simulink model "test_transfer_function"  (R2019b)
settings: Solver=ode4  StartTime=0.0  StopTime=100  FixedStep=1e-3  RelTol=1e-3
libraries: simulink x1
settings Model: Creator=bitgar  LastModifiedBy=bitgar
settings DataIOCC: ReturnWorkspaceOutputs=off

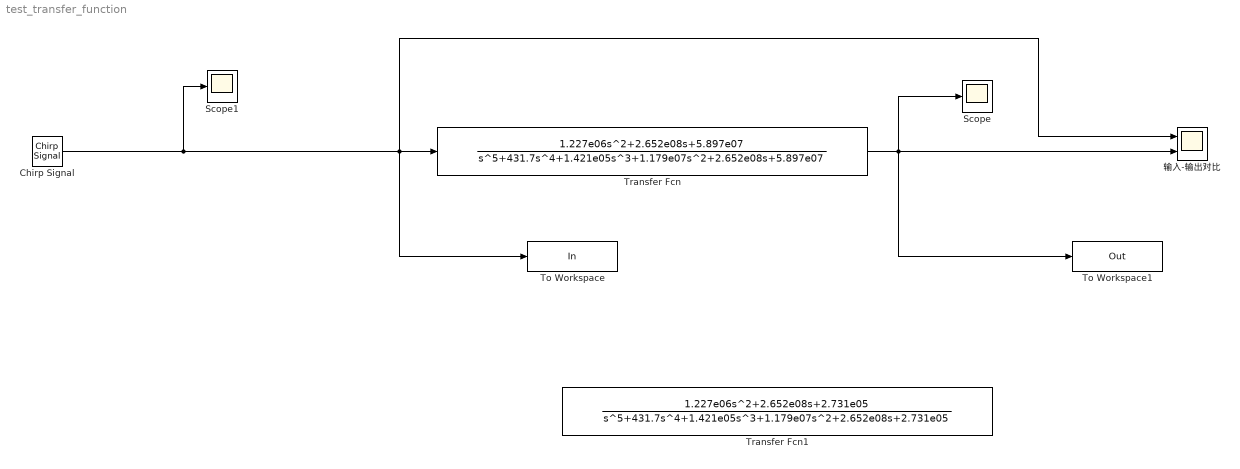
== system test_transfer_function ==
  Chirp Signal : simulink/Sources/Chirp Signal  f1=0.0001  T=400  f2=400
  Scope : Scope
  Scope1 : Scope
  To Workspace : ToWorkspace  VariableName=In  SampleTime=-1
  To Workspace1 : ToWorkspace  VariableName=Out  SampleTime=-1
  Transfer Fcn : TransferFcn  Numerator=[1.227e06 2.652e08 5.897e07]  Denominator=[1 431.7 1.421e05 1.179e07 2.652e08 5.897e07]
  Transfer Fcn1 : TransferFcn  Numerator=[1.227e06 2.652e08 2.731e05]  Denominator=[1 431.7 1.421e05 1.179e07 2.652e08 2.731e05]
  输入-输出对比 : Scope  NumInputPorts=2
  wires:
  Transfer Fcn/1 -> 输入-输出对比/2, To Workspace1/1, Scope/1
  Chirp Signal/1 -> Transfer Fcn/1, To Workspace/1, 输入-输出对比/1, Scope1/1
